simulink model "Full_Wave_Rectifier_HalfControlled_Rload_Quize_Diagram"  (R2018b)
settings: Solver=VariableStepAuto  StartTime=0.0  StopTime=0.06  RelTol=1e-3
libraries: powerlib x14
settings Model: Creator=A.hey  LastModifiedBy=A.hey

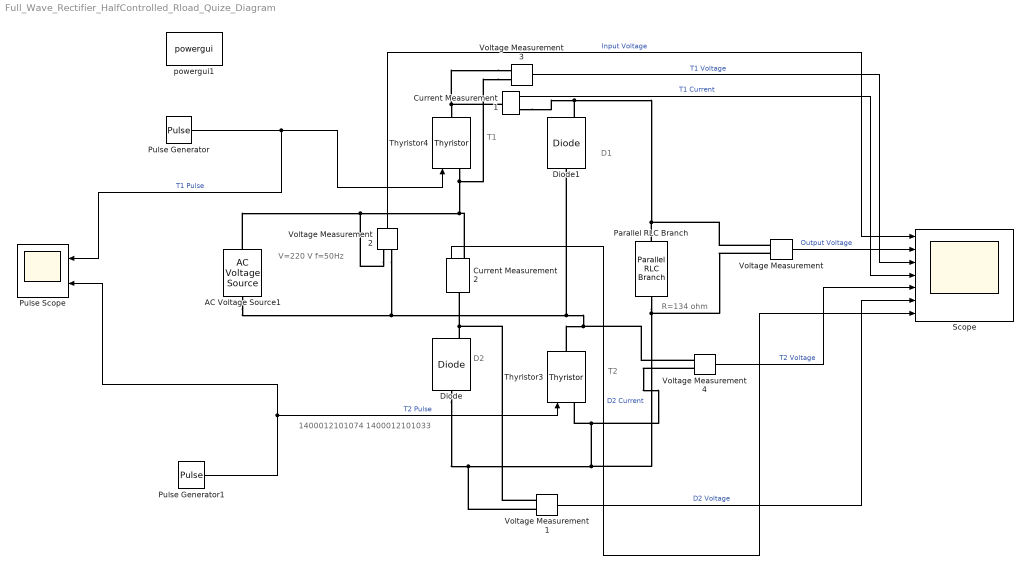
== system Full_Wave_Rectifier_HalfControlled_Rload_Quize_Diagram ==
  note: R=134 ohm
  note: D2
  note: 1400012101074
      | 1400012101033
  note: T1
  note: V=220 V
      | f=50Hz
  note: D1
  note: T2
  AC Voltage Source1 : powerlib/Electrical Sources/AC Voltage Source  Amplitude=220  Phase=0  Frequency=50  SampleTime=0  Measurements=None  BusType=swing  Pref=10e3  Qref=0  Qmin=-inf  Qmax=+inf
      settings: SourceProductName=Simscape Electrical
  Current Measurement1 : powerlib/Measurements/Current Measurement  PhasorSimulation=off  OutputType=Complex  PSBequivalent=0
      settings: SourceProductName=Simscape Electrical
  Current Measurement2 : powerlib/Measurements/Current Measurement  PhasorSimulation=off  OutputType=Complex  PSBequivalent=0
      settings: SourceProductName=Simscape Electrical
  Diode : powerlib/Power Electronics/Diode  Ron=0.001  Lon=0  Vf=0.8  IC=0  UseSnubber=0  Rs=500  Cs=250e-9  Measurements=on
  Diode1 : powerlib/Power Electronics/Diode  Ron=0.001  Lon=0  Vf=0.8  IC=0  UseSnubber=0  Rs=500  Cs=250e-9  Measurements=on
  Parallel RLC Branch : powerlib/Elements/Parallel RLC Branch  LConnTagsString=a  RConnTagsString=__new0  BranchType=R  Resistance=134  Inductance=1e-3  SetiL0=off  InitialCurrent=0  Capacitance=1e-6  Setx0=off  InitialVoltage=0  Measurements=None
      settings: SourceProductName=Simscape Electrical
  Pulse Generator : DiscretePulseGenerator  PulseType=Time based  Amplitude=10  Period=0.02  PulseWidth=50  PhaseDelay=0.005
  Pulse Generator1 : DiscretePulseGenerator  PulseType=Time based  Amplitude=10  Period=0.02  PulseWidth=25  PhaseDelay=0.005
  Pulse Scope : Scope  NumInputPorts=2
  "Scope " : Scope  NumInputPorts=7
  Thyristor3 : powerlib/Power Electronics/Thyristor  Ron=0.001  Lon=0  Vf=0.1  IC=0  Rs=500  Cs=250e-9  Measurements=off
      settings: SourceProductName=Simscape Electrical
  Thyristor4 : powerlib/Power Electronics/Thyristor  Ron=0.001  Lon=0  Vf=0.1  IC=0  Rs=500  Cs=250e-9  Measurements=off
      settings: SourceProductName=Simscape Electrical
  Voltage Measurement{,1..4} (5 alike) : powerlib/Measurements/Voltage Measurement  PhasorSimulation=off  OutputType=Complex  PSBequivalent=0
      settings: SourceProductName=Simscape Electrical
  powergui1 : powerlib/powergui  Priority=1  SimulationMode=Continuous  SampleTime=50e-6  frequency=60  Iterations=50  frequencyindice=50  Pbase=100e6  ErrMax=1e-4  UnitsV=kV  UnitsW=MW  buscounter=0  FunctionMessages=off  echomessages=off  EnableUseOfTLC=off  CurrentSourceSwitches=off  DisableSnubberDevices=off  DisableRonSwitches=off  DisableVfSwitches=off  DisplayEquations=off  SolverType=Tustin/Backward Euler (TBE)  Interpol=off  ExternalGateDelay=off  methode=off  Ts=100  x0status=blocks  SPID=on  SwTol=0  HookPort=off  RestoreLinks=warning  ResistiveCurrentMeasurement=off  Frange=[0:2:500]  Ylog=off  Xlog=on  ShowGrid=off  save=off  variable=ZData  structure=0  ZoomFFT=off  StartTime=0.0  cycles=1  DisplayStyle=1  fundamental=60  FreqAxis=off  MaxFrequency=1000  frequencyindicesteady=1  RmsSteady=1  display=off
  wires:
  Voltage Measurement/1 -> "Scope "/2  "Output Voltage"
  Pulse Generator/1 -> Pulse Scope/1, Thyristor4/1  "T1 Pulse"
  Voltage Measurement4/1 -> "Scope "/5  "T2 Voltage"
  Current Measurement2/1 -> "Scope "/7  "D2 Current"
  Current Measurement1/1 -> "Scope "/4  "T1 Current"
  Pulse Generator1/1 -> Thyristor3/1, Pulse Scope/2  "T2 Pulse"
  Voltage Measurement3/1 -> "Scope "/3  "T1 Voltage"
  Voltage Measurement1/1 -> "Scope "/6  "D2 Voltage"
  Voltage Measurement2/1 -> "Scope "/1  "Input Voltage"
  connections:
  Voltage Measurement3/LConn2 -- Current Measurement1/LConn1 -- Thyristor4/RConn1
  Voltage Measurement/LConn2 -- Parallel RLC Branch/RConn1 -- Thyristor3/LConn1 -- Voltage Measurement4/LConn1 -- Diode/LConn1 -- Voltage Measurement1/LConn1
  Voltage Measurement3/LConn1 -- Thyristor4/LConn1 -- AC Voltage Source1/RConn1 -- Voltage Measurement2/LConn1 -- Current Measurement2/RConn1
  Parallel RLC Branch/LConn1 -- Voltage Measurement/LConn1 -- Diode1/RConn1 -- Current Measurement1/RConn1
  Diode/RConn1 -- Voltage Measurement1/LConn2 -- Current Measurement2/LConn1
  AC Voltage Source1/LConn1 -- Thyristor3/RConn1 -- Voltage Measurement4/LConn2 -- Diode1/LConn1 -- Voltage Measurement2/LConn2
